simulink model "control1"  (R2015a)
settings: Solver=ode3  StartTime=0.0  StopTime=10.0  FixedStep=1/200  RelTol=1e-3
libraries: PoliArd x6
settings Model: ExtModeTrigDuration=2  Creator=User  LastModifiedBy=dell
settings OptimizationCC: OptimizeModelRefInitCode=on  LifeSpan=1
settings DebuggingCC: UnderspecifiedInitializationDetection=Classic  MergeDetectMultiDrivingBlocksExec=none
settings HardwareCC: ProdLargestAtomicInteger=Long  ProdLargestAtomicFloat=Double  ProdEndianess=LittleEndian  ProdHWDeviceType=ARM Compatible->ARM Cortex
settings RTWCC: SystemTargetFile=realtime.tlc  GenerateMakefile=off  TemplateMakefile=realtime.tmf  Description=Run on Target Hardware  RTWVerbose=off
settings ERTTargetCC: CombineOutputUpdateFcns=off  ExtModeTransport=3  ExtModeMexFile=ext_serial_win32_comm_rtt  ExtModeMexArgs=0 1 9600  ERTSrcFileBannerTemplate=realtime_code_template.cgt  ERTHdrFileBannerTemplate=realtime_code_template.cgt  ERTDataSrcFileTemplate=realtime_code_template.cgt  ERTDataHdrFileTemplate=realtime_code_template.cgt  ERTCustomFileTemplate=realtime_file_process.tlc

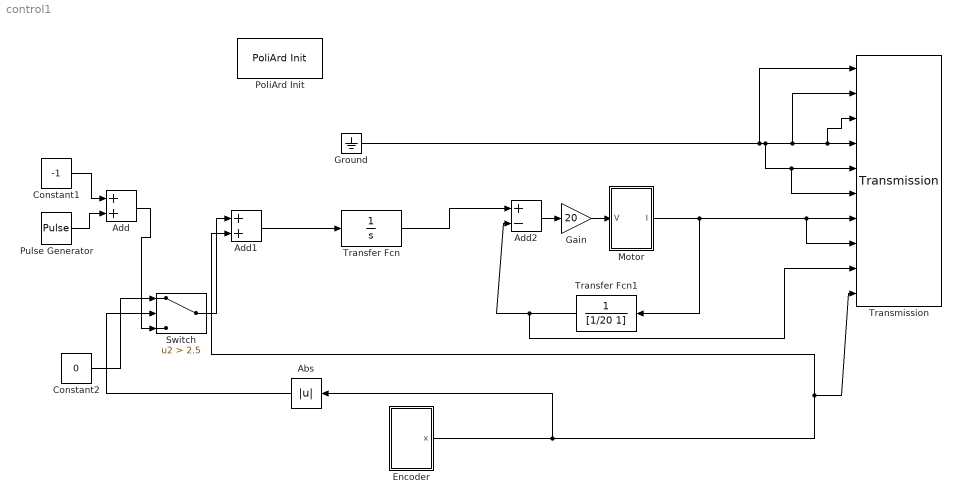
== system control1 ==
  Abs : Abs
  Add : Sum
  Add1 : Sum
  Add2 : Sum  Inputs=+-
  Constant1 : Constant  Value=-1
  Constant2 : Constant  Value=0
  "Encoder " : Subsystem
  Gain : Gain  Gain=20
  Ground : Ground
  Motor : Subsystem
  PoliArd Init : PoliArd/PoliArd Init
  Pulse Generator : DiscretePulseGenerator  PulseType=Time based  Period=20  PulseWidth=50
  Switch : Switch  Criteria=u2 > Threshold  Threshold=2.5
  Transfer Fcn : TransferFcn  Denominator=[1 0]
  Transfer Fcn1 : TransferFcn  Denominator=[1/20 1]
  Transmission : PoliArd/Transmission  sample_freq=200  sig_to_send=6
  wires:
  Ground/1 -> Transmission/1, Transmission/6, Transmission/5, Transmission/2, Transmission/3, Transmission/4
  Pulse Generator/1 -> Add/2
  Constant1/1 -> Add/1
  Add1/1 -> Transfer Fcn/1
  "Encoder "/1(x) -> Abs/1, Add1/2, Transmission/10
  Motor/1(I) -> Transfer Fcn1/1, Transmission/8, Transmission/7
  Transfer Fcn/1 -> Add2/1
  Transfer Fcn1/1 -> Transmission/9, Add2/2
  Gain/1 -> Motor/1(V)
  Add2/1 -> Gain/1
  Switch/1 -> Add1/1
  Abs/1 -> Switch/2
  Add/1 -> Switch/3
  Constant2/1 -> Switch/1

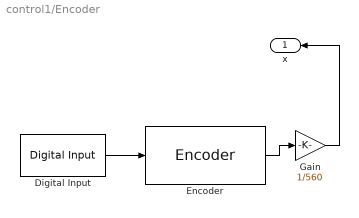
== system control1/Encoder  ==
  Digital Input : PoliArd/Digital Input  DI_pin=2  DIsample=1/200
  Encoder : PoliArd/Encoder  EncoderID=1  dt_enc=-1
  Gain : Gain  Gain=1/560
  x : Outport
  wires:
  Encoder/1 -> Gain/1
  Gain/1 -> x/1
  Digital Input/1 -> Encoder/1

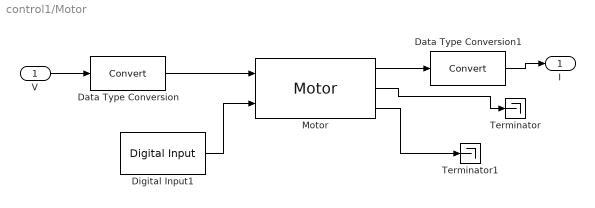
== system control1/Motor ==
  V : Inport
  Data Type Conversion : DataTypeConversion
  Data Type Conversion1 : DataTypeConversion
  Digital Input1 : PoliArd/Digital Input  DI_pin=3  DIsample=1/200
  Motor : PoliArd/Motor  MotorID=1  DC_bus_mask=12  dt_mot=1/200
  Terminator : Terminator
  Terminator1 : Terminator
  I : Outport
  wires:
  Data Type Conversion/1 -> Motor/1
  Digital Input1/1 -> Motor/2
  V/1 -> Data Type Conversion/1
  Motor/3 -> Terminator1/1
  Motor/2 -> Terminator/1
  Motor/1 -> Data Type Conversion1/1
  Data Type Conversion1/1 -> I/1
